simulink model "MOD_DEM_AM"  (R2024b)
settings: Solver=VariableStepAuto  StartTime=0.0  StopTime=1  RelTol=1e-3  EnableMultiTasking=on
libraries: dspfdesign x1
settings Model: Creator=Usuario  LastModifiedBy=RomaW11
settings SolverCC: AlgebraicLoopSolver=TrustRegion
settings DataIOCC: LimitDataPoints=on  ReturnWorkspaceOutputs=off
settings OptimizationCC: LifeSpan=inf
settings DebuggingCC: UnconnectedInputMsg=warning  UnconnectedOutputMsg=warning  UnconnectedLineMsg=warning  AllowSymbolicDim=off  SFUnexpectedBacktrackingDiag=warning  SFNoUnconditionalDefaultTransitionDiag=warning  SFExecutionAtInitializationDiag=none  ArithmeticOperatorsInVariantConditions=warning
settings ModelReferenceCC: EnableRefExpFcnMdlSchedulingChecks=on  PropagateSignalLabelsOutOfModel=off
settings SFSimCC: SimUseLocalCustomCode=off  CustomCodeUndefinedFunction=UseInterfaceOnly
settings RTWCC: RTWUseLocalCustomCode=off  GPUComputeCapability=3.5
settings CodeAppCC: StateflowObjectComments=on
settings GRTTargetCC: TargetLangStandard=C89/C90 (ANSI)
settings ConfigComp: CovMetricSettings=dw  CovSaveCumulativeToWorkspaceVar=on  CovSaveSingleToWorkspaceVar=on  CovExternalEMLEnable=off

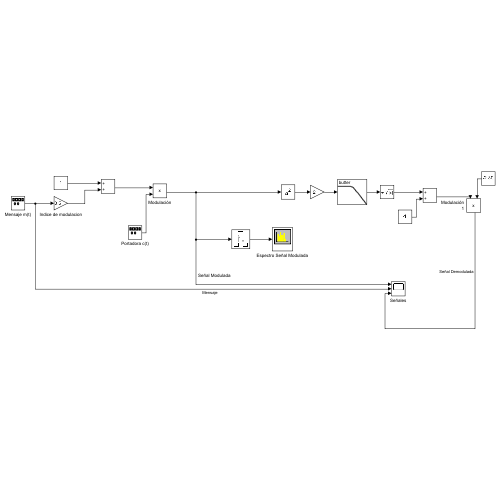
[thumbnail: Simulink's stored preview of the top-level diagram]
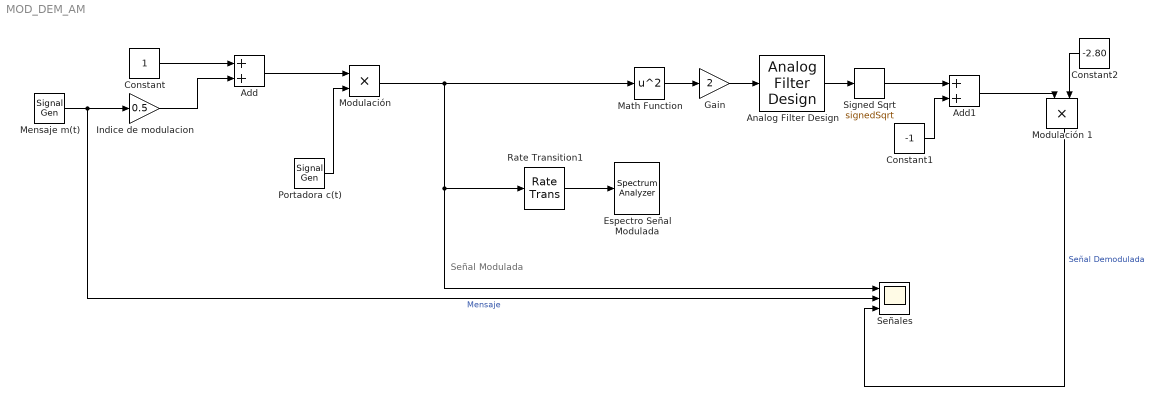
== system MOD_DEM_AM ==
  note: Señal Modulada
  Add : Sum
  Add1 : Sum
  Analog Filter Design : dspfdesign/Analog Filter Design  method=Butterworth  filttype=Lowpass  N=4  Wlo=2*pi*10000  Whi=80  Rp=2  Rs=40
  Constant : Constant
  Constant1 : Constant  Value=-1
  Constant2 : Constant  Value=-2.80
  Espectro Señal Modulada : SpectrumAnalyzer  WindowPosition=[312.000000,16.000000,1297.000000,1048.000000,]  ScopeFrameLocation=window  Method=Welch  SampleRate=1000000  AxesScaling=Manual  Span=1000000  StartFrequency=-500000  StopFrequency=500000  AveragingMethod=Running  YLabel=dBm  YLimits=[-111.39957098308905,31.069144841263995]  ShowGrid=off  AllowFFTLengthLessThanSamplesPerUpdate=on  DefaultConfigurationName=spbscopes.SpectrumAnalyzerBlockCfg
  Gain : Gain  Gain=2
  "Indice de modulacion " : Gain  Gain=0.5
  Math Function : Math  Operator=square  SignedPower=on
  "Mensaje m(t) " : SignalGenerator  Frequency=10000
  "Modulación " : Product
  Modulación 1 : Product
  "Portadora c(t) " : SignalGenerator  Frequency=50000
  Rate Transition1 : RateTransition  OutPortSampleTime=0.000001
  Señales : Scope  NumInputPorts=3
  Signed Sqrt : Sqrt  Operator=signedSqrt
  wires:
  Constant/1 -> Add/1
  "Portadora c(t) "/1 -> "Modulación "/2
  Add/1 -> "Modulación "/1
  "Modulación "/1 -> Señales/1, Rate Transition1/1, Math Function/1
  Rate Transition1/1 -> Espectro Señal Modulada/1
  Math Function/1 -> Gain/1
  Gain/1 -> Analog Filter Design/1
  Analog Filter Design/1 -> Signed Sqrt/1
  Signed Sqrt/1 -> Add1/1
  Constant1/1 -> Add1/2
  "Mensaje m(t) "/1 -> Señales/2, "Indice de modulacion "/1  "Mensaje"
  "Indice de modulacion "/1 -> Add/2
  Add1/1 -> Modulación 1/1
  Constant2/1 -> Modulación 1/2
  Modulación 1/1 -> Señales/3  "Señal Demodulada"
